simulink model "PUMA_8MM"  (Simulink 8.6)
settings: Solver=ode5  StartTime=0.0  StopTime=3  FixedStep=0.003  RelTol=1e-3
undefined symbols (not defined in the file): magnitude
libraries: vrlib x8, simulink x5
(part 2 of 2)

== matlab function BFT_old/PathFounder_ftk(tau) ==
  data: ksi output double; teta output double; fi output double; w input double; ax output double; ay output double; az output double; bx output double; by output double; bz output double; paramdt output double; paramSUM input double; time input double
function [ksi,teta,fi,ax,ay,az,bx,by,bz,paramdt] = fcn(w,paramSUM,time)

  % reset initial conditions, when -1 change on +1_
  
  % отсчет номера рабочего сплайна_
  num = 2;
  for k = 1:1:20
    if (paramSUM>k) num = k+2; end;
  end;
  param = paramSUM - num + 2;
  
  % =======================================================================
  
  %% задание опорных точек_
  % окружность_
  Pksi  = [0 0 0 0 0 0 0 0 0 0 0 0 0 0 0 0 0 0 0 0];
  Pteta = [0 0 0 0 0 0 0 0 0 0 0 0 0 0 0 0 0 0 0 0]; 
  Pfi   = [0 0 0 0 0 0 0 0 0 0 0 0 0 0 0 0 0 0 0 0];

  d = 0.4;%*1.525;
  b = 0.2*0;
  c = 0.2;
%  % окружность_
%  PN1ksi  = [d 0 -d 0 d 0 -d 0 d 0 -d 0 d 0 -d 0 d 0 -d 0];
%  PN1teta = [0 0 0 0 0 0 0 0 0 0 0 0 0 0 0 0 0 0 0 0];
%  PN1fi   = [0 -d 0 d 0 -d 0 d 0 -d 0 d 0 -d 0 d 0 -d 0 d];
%  PN2ksi  = [d 0 -d 0 d 0 -d 0 d 0 -d 0 d 0 -d 0 d 0 -d 0];
%  PN2teta = [0 0 0 0 0 0 0 0 0 0 0 0 0 0 0 0 0 0 0 0];
%  PN2fi   = [0 -d 0 d 0 -d 0 d 0 -d 0 d 0 -d 0 d 0 -d 0 d]; 

%  PN1ksi  = [0 0 0 0 0 0 0 0 0 0 0 0 0 0 0 0 0 0 0 0];
%  PN1teta = [0 0 0 0 0 0 0 0 0 0 0 0 0 0 0 0 0 0 0 0];
%  PN1fi   = [d -d d -d d -d d -d d -d d -d d -d d -d d -d d -d];
%  PN2ksi  = [0 0 0 0 0 0 0 0 0 0 0 0 0 0 0 0 0 0 0 0];
%  PN2teta = [0 0 0 0 0 0 0 0 0 0 0 0 0 0 0 0 0 0 0 0];
%  PN2fi   = [d -d d -d d -d d -d d -d d -d d -d d -d d -d d -d]; 

%  PN1ksi  = [0 0 0 0 0 0 0 0 0 0 0 0 0 0 0 0 0 0 0 0];
%  PN1teta = [d -d d -d d -d d -d d -d d -d d -d d -d d -d d -d];
%  PN1fi   = [0 0 0 0 0 0 0 0 0 0 0 0 0 0 0 0 0 0 0 0];
%  PN2ksi  = [0 0 0 0 0 0 0 0 0 0 0 0 0 0 0 0 0 0 0 0];
%  PN2teta = [d -d d -d d -d d -d d -d d -d d -d d -d d -d d -d];
%  PN2fi   = [0 0 0 0 0 0 0 0 0 0 0 0 0 0 0 0 0 0 0 0]; 

%  PN1ksi  = [d -d d -d d -d d -d d -d d -d d -d d -d d -d d -d];
%  PN1teta = [0 0 0 0 0 0 0 0 0 0 0 0 0 0 0 0 0 0 0 0];
%  PN1fi   = [0 0 0 0 0 0 0 0 0 0 0 0 0 0 0 0 0 0 0 0];
%  PN2ksi  = [d -d d -d d -d d -d d -d d -d d -d d -d d -d d -d];
%  PN2teta = [0 0 0 0 0 0 0 0 0 0 0 0 0 0 0 0 0 0 0 0];
%  PN2fi   = [0 0 0 0 0 0 0 0 0 0 0 0 0 0 0 0 0 0 0 0]; 

  PN1ksi  = [d -d d -d d -d d -d d -d d -d d -d d -d d -d d -d];
  PN1teta = [c -c c -c c -c c -c c -c c -c c -c c -c c -c c -c];
  PN1fi   = [-b b -b b -b b -b b -b b -b b -b b -b b -b b -b b];
  PN2ksi  = [d -d d -d d -d d -d d -d d -d d -d d -d d -d d -d];
  PN2teta = [c -c c -c c -c c -c c -c c -c c -c c -c c -c c -c];
  PN2fi   = [-b b -b b -b b -b b -b b -b b -b b -b b -b b -b b]; 

  % =======================================================================

  % расчет коэффициентов A,B,C,D_
  Aksi  = -Pksi(num)    + 3*PN1ksi(num)  - 3*PN2ksi(num)  + Pksi(num+1);
  Ateta = -Pteta(num)   + 3*PN1teta(num) - 3*PN2teta(num) + Pteta(num+1);
  Afi   = -Pfi(num)     + 3*PN1fi(num)   - 3*PN2fi(num)   + Pfi(num+1);
  Bksi  = 3*Pksi(num)   - 6*PN1ksi(num)  + 3*PN2ksi(num);
  Bteta = 3*Pteta(num)  - 6*PN1teta(num) + 3*PN2teta(num);
  Bfi   = 3*Pfi(num)    - 6*PN1fi(num)   + 3*PN2fi(num);
  Cksi  = -3*Pksi(num)  + 3*PN1ksi(num);
  Cteta = -3*Pteta(num) + 3*PN1teta(num);
  Cfi   = -3*Pfi(num)   + 3*PN1fi(num);
  Dksi  = Pksi(num);
  Dteta = Pteta(num);
  Dfi   = Pfi(num);
  
  ksi  = Aksi*param^3  + Bksi*param^2  + Cksi*param  + Dksi;
  teta = Ateta*param^3 + Bteta*param^2 + Cteta*param + Dteta;
  fi   = Afi*param^3   + Bfi*param^2   + Cfi*param   + Dfi;
  
ksi  = 0;
teta = 0;
fi   = 0;

  % расчет производной параметрического времени_
  paramdt = w/(  (Aksi*3*param^2+Bksi*2*param+Cksi)^2 + (Ateta*3*param^2+Bteta*2*param+Cteta)^2 + (Afi*3*param^2+Bfi*2*param+Cfi)^2  )^(0.5);

  % =======================================================================
  
  Ea = [ 0 ; 1 ; 0 ];
  Eb = [ 0 ; 0 ; 1 ];
  
  % Mx(ksi) - поворот вокруг оси OX на на угол ksi_
  Mxksi  = [ 1         0          0         ; 0       cos(ksi) (-sin(ksi)) ; 0            sin(ksi) cos(ksi) ];
  Myteta = [ cos(teta) 0          sin(teta) ; 0       1        0           ; (-sin(teta)) 0        cos(teta)];
  Mzfi   = [ cos(fi)   (-sin(fi)) 0         ; sin(fi) cos(fi)  0           ; 0            0        1        ];  
  
  a = Mxksi*Myteta*Mzfi*Ea;
  b = Mxksi*Myteta*Mzfi*Eb;
  
  ax = a(1,1);
  ay = a(2,1);
  az = a(3,1);
  bx = b(1,1);
  by = b(2,1);
  bz = b(3,1);
  
%ax = 0;
%az = 0.2*sin(time*3.141592);
%ay = sqrt(1-az*az);
%bx = 0;
%by = 0.2*sin(time*3.141592);
%bz = sqrt(1-by*by); 

%ax = 0;
%ay = 0;
%az = 1;
%bx = -1;
%by = 0;
%bz = 0;

end

== matlab function BFq7_integrator/OZK_q7+ ==
  data: x input double; y input double; z input double; q7pr output double; ax input double; ay input double; az input double; bx input double; by input double; bz input double; q7 input double; o1 output double; o2 output double; o3 output double
function [q7pr,o1,o2,o3] = fcn(x,y,z,ax,ay,az,bx,by,bz,q7)
   
   % q7 настраивается так, чтобы расстояние W2_cr-W2 было больше Rmin.
 
    pi = 3.14159265358979;
    % Длины звеньев.
    L1 = 0.4;
    L2 = 0.7;
    L3 = 0.7;
    L4 = 0.1;

    % Тестовая надбавка для q7.
    dq = 0.01;
    
    % Ограничения по положению по степеням подвижности i=1,7.
    q1min = -pi/2;    q1max =  pi/2;
    q2min = -pi/2;    q2max =  pi/2;
    q3min = -pi/2;    q3max =  pi/2;
    q4min = -pi/2;    q4max =  pi/2;
    q5min = -pi/2;    q5max =  pi/2;
    q6min = -pi/2;    q6max =  pi/2;
    q7min = -5;       q7max =  5;
    
% =========================================================================    
% ===================== Опред. текущее значение q1-q6 =====================  
% =========================================================================

    rx = x - q7;
    ry = y     ;
    rz = z     ;

    Rx = rx-ax*L4;
    Ry = ry-ay*L4;
    Rz = rz-az*L4;
 
  if (Ry==0) Ry = 0.0000001; end;  
  q1 = -atan(Rx/Ry);
  
    f1 = (Rz-L1)/L3;
    f2 = -L2/L3;
    f3 = Ry/(L3*cos(q1));
    
    g1 = 2*f1*f2;
    g2 = 2*f2*f3;
    g3 = 1-f1*f1-f2*f2-f3*f3;
           
  q2 = asin(g3/sqrt(g1*g1+g2*g2)) - atan(f3/f1); 
    if (q2<-pi/2) q2 = q2+pi; end;
  q3 = asin(f1+f2*sin(q2)) - q2;   
  
    fi  = q2+q3;  
    sfi = sin(fi);
    cfi = cos(fi);
    if (ay==0) ay = 0.0000001; end;  
    alfa = -q1 - atan(ax/ay); 
    if (abs(alfa)<0.0000001) alfa = 0; end;

  if (alfa >= 0) q5 =  acos(-ax*sin(q1)*cfi + ay*cos(q1)*cfi + az*sfi); 
  else           q5 = -acos(-ax*sin(q1)*cfi + ay*cos(q1)*cfi + az*sfi);
  end;                                                                 
  
    k = az - sfi*cos(q5);

  if (q5==0) q5 = 0.0000001; end;
  q4 = acos((-ax*cos(q1)-ay*sin(q1))/sin(q5));
  if (k  < 0) q4 = -q4; end; 
  if (q5 < 0) q4 = -q4; end; 
    
    gammax =  bz*(sin(q1)*sin(q4) - cos(q1)*sfi*cos(q4)) - by*cfi*cos(q4);
    gammay = -bz*(cos(q1)*sin(q4) + sin(q1)*sfi*cos(q4)) + bx*cfi*cos(q4);
    
    betta = gammax*ax + gammay*ay;
    
  q6 = acos(  bx*(cos(q1)*sin(q4)+sin(q1)*sfi*cos(q4))  +  by*(sin(q1)*sin(q4)-cos(q1)*sfi*cos(q4))  +  bz*(cfi*cos(q4))  );
  if (betta<0)  q6 = -q6; end; 
  
% -------------------- Текущее значение maxInd --------------------------

  Ind1  = abs(q1)/q1max;
  Ind2  = abs(q2)/q2max;
  Ind3  = abs(q3)/q3max;
  Ind4  = abs(q4)/q4max;
  Ind5  = abs(q5)/q5max;
  Ind6  = abs(q6)/q6max;
  Ind7  = abs(q7)/q7max;
  Ind8  = ( 2 - sqrt(ax*ax+ay*ay) - sqrt(rx*rx+ry*ry)/(L2+L3+L4) ) / 2;
  Ind9  = ( q5max - abs(q5) )/ q5max;
  Ind10 = ( q3max - abs(q3)/2.5 )/ q3max; % 4.7
  
  J = 0;
  J = max (J,Ind1);
  J = max (J,Ind2);
  J = max (J,Ind3);
  J = max (J,Ind4);
  J = max (J,Ind5);
  J = max (J,Ind6);
  J = max (J,Ind7);
  J = max (J,Ind8);
  J = max (J,Ind9);
  J = max (J,Ind10);

  maxInd = J;
  
% =========================================================================    
% ============================ @'но для q7+dq =============================  
% ========================================================================= 

    rx = x - (q7+dq);
    ry = y          ;
    rz = z          ;

    Rx = rx-ax*L4;
    Ry = ry-ay*L4;
    Rz = rz-az*L4;
 
  if (Ry==0) Ry = 0.0000001; end;  
  q1 = -atan(Rx/Ry);
  
    f1 = (Rz-L1)/L3;
    f2 = -L2/L3;
    f3 = Ry/(L3*cos(q1));
    
    g1 = 2*f1*f2;
    g2 = 2*f2*f3;
    g3 = 1-f1*f1-f2*f2-f3*f3;
           
  q2 = asin(g3/sqrt(g1*g1+g2*g2)) - atan(f3/f1); 
    if (q2<-pi/2) q2 = q2+pi; end;
  q3 = asin(f1+f2*sin(q2)) - q2;   
  
    fi  = q2+q3;  
    sfi = sin(fi);
    cfi = cos(fi);
    if (ay==0) ay = 0.0000001; end;  
    alfa = -q1 - atan(ax/ay); 
    if (abs(alfa)<0.0000001) alfa = 0; end;

  if (alfa >= 0) q5 =  acos(-ax*sin(q1)*cfi + ay*cos(q1)*cfi + az*sfi); 
  else           q5 = -acos(-ax*sin(q1)*cfi + ay*cos(q1)*cfi + az*sfi);
  end;                                                                 
  
    k = az - sfi*cos(q5);

  if (q5==0) q5 = 0.0000001; end;
  q4 = acos((-ax*cos(q1)-ay*sin(q1))/sin(q5));
  if (k  < 0) q4 = -q4; end; 
  if (q5 < 0) q4 = -q4; end; 
    
    gammax =  bz*(sin(q1)*sin(q4) - cos(q1)*sfi*cos(q4)) - by*cfi*cos(q4);
    gammay = -bz*(cos(q1)*sin(q4) + sin(q1)*sfi*cos(q4)) + bx*cfi*cos(q4);
    
    betta = gammax*ax + gammay*ay;
    
  q6 = acos(  bx*(cos(q1)*sin(q4)+sin(q1)*sfi*cos(q4))  +  by*(sin(q1)*sin(q4)-cos(q1)*sfi*cos(q4))  +  bz*(cfi*cos(q4))  );
  if (betta<0)  q6 = -q6; end; 
  
% -------------------- Текущее значение maxInd(q7+dq7) --------------------

  Ind1  = abs(q1)/q1max;
  Ind2  = abs(q2)/q2max;
  Ind3  = abs(q3)/q3max;
  Ind4  = abs(q4)/q4max;
  Ind5  = abs(q5)/q5max;
  Ind6  = abs(q6)/q6max;
  Ind7  = abs(q7)/q7max;
  Ind8  = ( 2 - sqrt(ax*ax+ay*ay) - sqrt(rx*rx+ry*ry)/(L2+L3+L4) ) / 2;
  Ind9  = ( q5max - abs(q5) )/ q5max;
  Ind10 = ( q3max - abs(q3)/2.5 )/ q3max; % 4.7
  
  J = 0;
  J = max (J,Ind1);
  J = max (J,Ind2);
  J = max (J,Ind3);
  J = max (J,Ind4);
  J = max (J,Ind5);
  J = max (J,Ind6);
  J = max (J,Ind7);
  J = max (J,Ind8);
  J = max (J,Ind9);
  J = max (J,Ind10);

  maxIndp = J;
         
% =========================================================================    
% ============================ @'но для q7-dq =============================   
% =========================================================================
   
    rx = x - (q7-dq);
    ry = y          ;
    rz = z          ;

    Rx = rx-ax*L4;
    Ry = ry-ay*L4;
    Rz = rz-az*L4;
 
  if (Ry==0) Ry = 0.0000001; end;  
  q1 = -atan(Rx/Ry);
  
    f1 = (Rz-L1)/L3;
    f2 = -L2/L3;
    f3 = Ry/(L3*cos(q1));
    
    g1 = 2*f1*f2;
    g2 = 2*f2*f3;
    g3 = 1-f1*f1-f2*f2-f3*f3;
           
  q2 = asin(g3/sqrt(g1*g1+g2*g2)) - atan(f3/f1); 
    if (q2<-pi/2) q2 = q2+pi; end;
  q3 = asin(f1+f2*sin(q2)) - q2;   
  
    fi  = q2+q3;  
    sfi = sin(fi);
    cfi = cos(fi);
    if (ay==0) ay = 0.0000001; end;  
    alfa = -q1 - atan(ax/ay); 
    if (abs(alfa)<0.0000001) alfa = 0; end;

  if (alfa >= 0) q5 =  acos(-ax*sin(q1)*cfi + ay*cos(q1)*cfi + az*sfi); 
  else           q5 = -acos(-ax*sin(q1)*cfi + ay*cos(q1)*cfi + az*sfi);
  end;                                                                 
  
    k = az - sfi*cos(q5);

  if (q5==0) q5 = 0.00001; end;
  q4 = acos((-ax*cos(q1)-ay*sin(q1))/sin(q5));
  if (k  < 0) q4 = -q4; end; 
  if (q5 < 0) q4 = -q4; end; 
    
    gammax =  bz*(sin(q1)*sin(q4) - cos(q1)*sfi*cos(q4)) - by*cfi*cos(q4);
    gammay = -bz*(cos(q1)*sin(q4) + sin(q1)*sfi*cos(q4)) + bx*cfi*cos(q4);
    
    betta = gammax*ax + gammay*ay;
    
  q6 = acos(  bx*(cos(q1)*sin(q4)+sin(q1)*sfi*cos(q4))  +  by*(sin(q1)*sin(q4)-cos(q1)*sfi*cos(q4))  +  bz*(cfi*cos(q4))  );
  if (betta<0)  q6 = -q6; end; 
  
% -------------------- Текущее значение maxInd(q7-dq7) --------------------

  Ind1  = abs(q1)/q1max;
  Ind2  = abs(q2)/q2max;
  Ind3  = abs(q3)/q3max;
  Ind4  = abs(q4)/q4max;
  Ind5  = abs(q5)/q5max;
  Ind6  = abs(q6)/q6max;
  Ind7  = abs(q7)/q7max;
  Ind8  = ( 2 - sqrt(ax*ax+ay*ay) - sqrt(rx*rx+ry*ry)/(L2+L3+L4) ) / 2;
  Ind9  = ( q5max - abs(q5) )/ q5max;
  Ind10 = ( q3max - abs(q3)/2.5 )/ q3max; % 4.7
  
  J = 0;
  J = max (J,Ind1);
  J = max (J,Ind2);
  J = max (J,Ind3);
  J = max (J,Ind4);
  J = max (J,Ind5);
  J = max (J,Ind6);
  J = max (J,Ind7);
  J = max (J,Ind8);
  J = max (J,Ind9);
  J = max (J,Ind10);

  maxIndn = J;
  
% =========================================================================    
% ============================= Выбор q7pr +/- ============================  
% =========================================================================  

  % q7pr - фиксированная скорость перемещения основания робота. 
  q7pr = 0.3;
  % Indth - пороговое значение максимального индикатора. 
  Indth = 0.9;

  if (maxIndn<maxIndp) q7pr = -q7pr; end;
  if (maxInd <Indth)   q7pr = 0;     end;

  o1 = maxInd;
  o2 = maxIndp;
  o3 = maxIndn;
  
end

== matlab function BFT_old/PathFounder_xyz(tau) ==
  data: v input double; x output double; y output double; z output double; num output double; paramdt output double; paramSUM input double
function [x,y,z,num,paramdt] = fcn(v,paramSUM)

  % reset initial conditions, when -1 change on +1.
  
  % Отсчет номера рабочего сплайна.
  num = 2;
  for k = 1:1:99
    if (paramSUM>k) num = k+2; end;
  end;
  param = paramSUM - num + 2;
  
  L1 = 0.4;
  L2 = 0.7;
  L3 = 0.7;
  L4 = 0.1;  
  
  % =======================================================================
  
  %% Окружность 0.4R с центром в (.)(0;ky;kz), наклоненная в пространстве.
%  ky = 1.1;   % смещение по оси оу.                                    
%  kz = 0.5;   % смещение по оси оz.
%  R  = 0.35;  % радиус окружности. 
%  fi = -0.2;  % угол наклона окружности.
%    dy00 = 0; % смещения окружности по оси оу.
%    dy05 = 0.5*R*sin(-fi); 
%    dy10 = 1.0*R*sin(-fi);
%    dy15 = 1.5*R*sin(-fi);
%    dy20 = 2.0*R*sin(-fi);
%  Px = [0       R       0       -R      0       R       0       -R      0       R       0       -R      0       R       0       -R      0       R       0       -R      ];
%  Py = [ky+dy00 ky+dy10 ky+dy20 ky+dy10 ky+dy00 ky+dy10 ky+dy20 ky+dy10 ky+dy00 ky+dy10 ky+dy20 ky+dy10 ky+dy00 ky+dy10 ky+dy20 ky+dy10 ky+dy00 ky+dy10 ky+dy20 ky+dy10 ]; 
%  Pz = [kz-R    kz      kz+R    kz      kz-R    kz      kz+R    kz      kz-R    kz      kz+R    kz      kz-R    kz      kz+R    kz      kz-R    kz      kz+R    kz      ];
  % Направляющие.
%  d = 0.02075*R/0.4;
%  PN1x = [R/2+d    R        -R/2-d    -R       R/2+d    R        -R/2-d    -R       R/2+d    R        -R/2-d    -R       R/2+d    R        -R/2-d    -R       R/2+d    R        -R/2-d    -R       ];
%  PN1y = [ky+dy00  ky+dy15  ky+dy20   ky+dy05  ky+dy00  ky+dy15  ky+dy20   ky+dy05  ky+dy00  ky+dy15  ky+dy20   ky+dy05  ky+dy00  ky+dy15  ky+dy20   ky+dy05  ky+dy00  ky+dy15  ky+dy20   ky+dy05  ];
%  PN1z = [kz-R     kz+R/2+d kz+R      kz-R/2-d kz-R     kz+R/2+d kz+R      kz-R/2-d kz-R     kz+R/2+d kz+R      kz-R/2-d kz-R     kz+R/2+d kz+R      kz-R/2-d kz-R     kz+R/2+d kz+R      kz-R/2-d ];
%  PN2x = [R        R/2+d    -R        -R/2-d   R        R/2+d    -R        -R/2-d   R        R/2+d    -R        -R/2-d   R        R/2+d    -R        -R/2-d   R        R/2+d    -R        -R/2-d   ];
%  PN2y = [ky+dy05  ky+dy20  ky+dy15   ky+dy00  ky+dy05  ky+dy20  ky+dy15   ky+dy00  ky+dy05  ky+dy20  ky+dy15   ky+dy00  ky+dy05  ky+dy20  ky+dy15   ky+dy00  ky+dy05  ky+dy20  ky+dy15   ky+dy00  ];
%  PN2z = [kz-R/2-d kz+R     kz+R/2+d  kz-R     kz-R/2-d kz+R     kz+R/2+d  kz-R     kz-R/2-d kz+R     kz+R/2+d  kz-R     kz-R/2-d kz+R     kz+R/2+d  kz-R     kz-R/2-d kz+R     kz+R/2+d  kz-R     ]; 

  %% Синусоида y=A*sin(...)+c
%  A  = 0.05;  % амплитуда в плоскости OXY.
%  B  = 0.25;  % амплитуда в плоскости OXZ.
%  c  = 1.2;   % смещение по оси OY.
%  k  = 0.4;   % смещение по оси OZ.
%  L  = 0.15;  % растягивание по OX.
%  Px = [-4*L -3*L  -2*L  -1*L   0*L   1*L   2*L   3*L   4*L   5*L   6*L   7*L   8*L   9*L   10*L  11*L  12*L  13*L  14*L  15*L ];
%  Py = [c    c     c     c      c     c     c     c     c     c     c     c     c     c     c     c     c     c     c     c    ];
%  Pz = [k    k     k     k      k     k     k     k     k     k     k     k     k     k     k     k     k     k     k     k    ];    
  % Направляющие.
%  d = 0.05;  % смещение направляющих.
%  PN1x = [-4*L+d -3*L+d -2*L+d -1*L+d 0*L+d 1*L+d 2*L+d 3*L+d 4*L+d 5*L+d 6*L+d 7*L+d 8*L+d 9*L+d  10*L+d 11*L+d 12*L+d 13*L+d 14*L+d 15*L+d];
%  PN1y = [c+A    c-A    c+A    c-A    c+A   c-A   c+A   c-A   c+A   c-A   c+A   c-A   c+A   c-A    c+A    c-A    c+A    c-A    c+A    c-A   ];
%  PN1z = [k+B    k-B    k+B    k-B    k+B   k-B   k+B   k-B   k+B   k-B   k+B   k-B   k+B   k-B    k+B    k-B    k+B    k-B    k+B    k-B   ]; 
%  PN2x = [-3*L-d -2*L-d -1*L-d 0*L-d  1*L-d 2*L-d 3*L-d 4*L-d 5*L-d 6*L-d 7*L-d 8*L-d 9*L-d 10*L-d 11*L-d 12*L-d 13*L-d 14*L-d 15*L-d 16*L-d];
%  PN2y = [c+A    c-A    c+A    c-A    c+A   c-A   c+A   c-A   c+A   c-A   c+A   c-A   c+A   c-A    c+A    c-A    c+A    c-A    c+A    c-A   ];
%  PN2z = [k+B    k-B    k+B    k-B    k+B   k-B   k+B   k-B   k+B   k-B   k+B   k-B   k+B   k-B    k+B    k-B    k+B    k-B    k+B    k-B   ];  

  %% Кривая, поднимающейся снизу вверх по поверхности цилиндра радиусом R и высотой H. 
  %   важны только первые 5 сплайнов.
%  R = 0.7;  % радиус цилиндра.
%  H = 0.25; % коэффициент высоты цилиндра.
%  Px = [0*R  1*R 0*R -1*R 0*R  0*R  1*R 0*R -1*R 0*R  0*R  1*R 0*R -1*R 0*R  0*R  1*R 0*R -1*R 0*R  ];
%  Py = [-1*R 0*R 1*R 0*R  -1*R -1*R 0*R 1*R 0*R  -1*R -1*R 0*R 1*R 0*R  -1*R -1*R 0*R 1*R 0*R  -1*R ]; 
%  Pz = [-1*H 0*H 1*H 2*H  3*H  -1*H 0*H 1*H 2*H  3*H  -1*H 0*H 1*H 2*H  3*H  -1*H 0*H 1*H 2*H  3*H  ];   
  % Направляющие.
%  d = 0.02075*2.5*R;
%  PN1x = [0.5*R+d     1*R        -0.5*R-d   -1*R      0.5*R+d     0.5*R+d     1*R        -0.5*R-d   -1*R      0.5*R+d     0.5*R+d     1*R        -0.5*R-d   -1*R      0.5*R+d     0.5*R+d     1*R        -0.5*R-d   -1*R      0.5*R+d     ];
%  PN1y = [-1*R        0.5*R+d    1*R        -0.5*R-d  -1*R        -1*R        0.5*R+d    1*R        -0.5*R-d  -1*R        -1*R        0.5*R+d    1*R        -0.5*R-d  -1*R        -1*R        0.5*R+d    1*R        -0.5*R-d  -1*R        ];
%  PN1z = [-0.75*H+d/5 0.25*H+d/5 1.25*H+d/5 2.25*H+d/5 3.25*H+d/5 -0.75*H+d/5 0.25*H+d/5 1.25*H+d/5 2.25*H+d/5 3.25*H+d/5 -0.75*H+d/5 0.25*H+d/5 1.25*H+d/5 2.25*H+d/5 3.25*H+d/5 -0.75*H+d/5 0.25*H+d/5 1.25*H+d/5 2.25*H+d/5 3.25*H+d/5 ];
%  PN2x = [1*R         0.5*R+d    -1*R       -0.5*R-d  1*R         1*R         0.5*R+d    -1*R       -0.5*R-d  1*R         1*R         0.5*R+d    -1*R       -0.5*R-d  1*R         1*R         0.5*R+d    -1*R       -0.5*R-d  1*R         ];
%  PN2y = [-0.5*R-d    1*R        0.5*R+d    -1*R      -0.5*R-d    -0.5*R-d    1*R        0.5*R+d    -1*R      -0.5*R-d    -0.5*R-d    1*R        0.5*R+d    -1*R      -0.5*R-d    -0.5*R-d    1*R        0.5*R+d    -1*R      -0.5*R-d    ];
%  PN2z = [-0.25*H-d/5 0.75*H-d/5 1.75*H-d/5 2.75*H-d/5 3.75*H-d/5 -0.25*H-d/5 0.75*H-d/5 1.75*H-d/5 2.75*H-d/5 3.75*H-d/5 -0.25*H-d/5 0.75*H-d/5 1.75*H-d/5 2.75*H-d/5 3.75*H-d/5 -0.25*H-d/5 0.75*H-d/5 1.75*H-d/5 2.75*H-d/5 3.75*H-d/5 ]; 

  %% Прямая, параллельная oz, проходящая через (X;Y;Z).
%  X = 0;
%  Y = 1.1;
%  Z = 1;
%  Px = [X   X      X     X      X   X   X      X     X      X   X   X      X     X      X   X   X      X     X      X   ];
%  Py = [Y   Y      Y     Y      Y   Y   Y      Y     Y      Y   Y   Y      Y     Y      Y   Y   Y      Y     Y      Y   ];
%  Pz = [1*Z 0.75*Z 0.5*Z 0.25*Z 0*Z 1*Z 0.75*Z 0.5*Z 0.25*Z 0*Z 1*Z 0.75*Z 0.5*Z 0.25*Z 0*Z 1*Z 0.75*Z 0.5*Z 0.25*Z 0*Z ]; 
  % Направляющие.
%  PN1x = [X      X      X      X      X       X      X      X      X      X       X      X      X      X      X       X      X      X      X      X       ];
%  PN1y = [Y      Y      Y      Y      Y       Y      Y      Y      Y      Y       Y      Y      Y      Y      Y       Y      Y      Y      Y      Y       ];
%  PN1z = [0.95*Z 0.70*Z 0.45*Z 0.20*Z -0.05*Z 0.95*Z 0.70*Z 0.45*Z 0.20*Z -0.05*Z 0.95*Z 0.70*Z 0.45*Z 0.20*Z -0.05*Z 0.95*Z 0.70*Z 0.45*Z 0.20*Z -0.05*Z ];
%  PN2x = [X      X      X      X      X       X      X      X      X      X       X      X      X      X      X       X      X      X      X      X       ];
%  PN2y = [Y      Y      Y      Y      Y       Y      Y      Y      Y      Y       Y      Y      Y      Y      Y       Y      Y      Y      Y      Y       ];
%  PN2z = [0.80*Z 0.55*Z 0.30*Z 0.05*Z -0.20*Z 0.80*Z 0.55*Z 0.30*Z 0.05*Z -0.20*Z 0.80*Z 0.55*Z 0.30*Z 0.05*Z -0.20*Z 0.80*Z 0.55*Z 0.30*Z 0.05*Z -0.20*Z ];

  %% Эллипс. Поперечные сечения - L и W.
%  L = 0.5;
%  W = 2;
%  Px = [-L L -L L -L L -L L -L L -L L -L L -L L -L L -L L];
%  Py = [0  0 0  0 0  0 0  0 0  0 0  0 0  0 0  0 0  0 0  0]; 
%  Pz = [0  0 0  0 0  0 0  0 0  0 0  0 0  0 0  0 0  0 0  0];  
  % Направляющие.
%  PN1x = [-L L  -L L  -L L  -L L  -L L  -L L  -L L  -L L  -L L  -L L ];
%  PN1y = [W  -W W  -W W  -W W  -W W  -W W  -W W  -W W  -W W  -W W  -W];
%  PN1z = [0  0  0  0  0  0  0  0  0  0  0  0  0  0  0  0  0  0  0  0 ];
%  PN2x = [L  -L L  -L L  -L L  -L L  -L L  -L L  -L L  -L L  -L L  -L];
%  PN2y = [W  -W W  -W W  -W W  -W W  -W W  -W W  -W W  -W W  -W W  -W];
%  PN2z = [0  0  0  0  0  0  0  0  0  0  0  0  0  0  0  0  0  0  0  0 ];

  %% Хитрые спирали.
%  L = 0.15;   % растягивание по ox.
%  H = 1.1;    % смещение по oy.
%  J = 0.25;   % смещение по oz.
%  M = 0.3;    % ширина петель.
%  k = 0.2;    % растягивание петель.
%  Px = [-4*L -3*L  -2*L  -1*L   0*L   1*L   2*L   3*L   4*L   5*L   6*L   7*L   8*L   9*L   10*L  11*L  12*L  13*L  14*L  15*L ];
%  Py = [H     H     H     H     H     H     H     H     H     H     H     H     H     H     H     H     H     H     H     H    ];
%  Pz = [J     J     J     J     J     J     J     J     J     J     J     J     J     J     J     J     J     J     J     J    ]; 
  % Направляющие.
%  PN1x = [-3*L+k  -2*L+k  -1*L+k  0*L+k   1*L+k   2*L+k   3*L+k   4*L+k   5*L+k   6*L+k   7*L+k   8*L+k   9*L+k   10*L+k  11*L+k  12*L+k  13*L+k  14*L+k  15*L+k  16*L+k  ];
%  PN1y = [H       H       H       H       H       H       H       H       H       H       H       H       H       H       H       H       H       H       H       H       ];
%  PN1z = [J+M     J-M     J+M     J-M     J+M     J-M     J+M     J-M     J+M     J-M     J+M     J-M     J+M     J-M     J+M     J-M     J+M     J-M     J+M     J-M     ];
%  PN2x = [-4*L-k  -3*L-k  -2*L-k  -1*L-k  0*L-k   1*L-k   2*L-k   3*L-k   4*L-k   5*L-k   6*L-k   7*L-k   8*L-k   9*L-k   10*L-k  11*L-k  12*L-k  13*L-k  14*L-k  15*L-k  ];
%  PN2y = [H       H       H       H       H       H       H       H       H       H       H       H       H       H       H       H       H       H       H       H       ];
%  PN2z = [J+M     J-M     J+M     J-M     J+M     J-M     J+M     J-M     J+M     J-M     J+M     J-M     J+M     J-M     J+M     J-M     J+M     J-M     J+M     J-M     ];

  %% Прямая, параллельная ox, проходящая через (X;Y;Z).
%  X  = 0.3;
%  Y  = L2*cos(pi/6)+L3+L4*0.97;
%  Z  = L1+L2*sin(pi/6);
%  Px = [-1*X -0.75*X -0.5*X -0.25*X 0*X 0.25*X 0.5*X 0.75*X 1*X 0.75*X 0.5*X 0.25*X 0*X -0.25*X -0.5*X -0.75*X -1*X -0.75*X -0.5*X -0.25*X ];
%  Py = [Y    Y       Y      Y       Y   Y      Y     Y      Y   Y      Y     Y      Y   Y       Y      Y       Y    Y       Y      Y       ];
%  Pz = [Z    Z       Z      Z       Z   Z      Z     Z      Z   Z      Z     Z      Z   Z       Z      Z       Z    Z       Z      Z       ];
  % Направляющие.
%  PN1x = [-0.9*X -0.7*X -0.4*X -0.2*X 0.1*X  0.3*X 0.6*X 0.8*X 0.9*X 0.7*X 0.4*X 0.2*X -0.1*X -0.3*X -0.6*X -0.8*X -0.9*X -0.7*X -0.4*X -0.2*X ];
%  PN1y = [Y      Y      Y      Y      Y      Y     Y     Y     Y     Y     Y     Y     Y      Y      Y      Y      Y      Y      Y      Y      ];
%  PN1z = [Z      Z      Z      Z      Z      Z     Z     Z     Z     Z     Z     Z     Z      Z      Z      Z      Z      Z      Z      Z      ];
%  PN2x = [-0.8*X -0.6*X -0.3*X -0.1*X 0.2*X  0.4*X 0.7*X 0.9*X 0.8*X 0.6*X 0.3*X 0.1*X -0.2*X -0.4*X -0.7*X -0.9*X -0.8*X -0.6*X -0.3*X -0.1*X ];
%  PN2y = [Y      Y      Y      Y      Y      Y     Y     Y     Y     Y     Y     Y     Y      Y      Y      Y      Y      Y      Y      Y      ];
%  PN2z = [Z      Z      Z      Z      Z      Z     Z     Z     Z     Z     Z     Z     Z      Z      Z      Z      Z      Z      Z      Z      ];

  %% Окружность 0.4R с центром в (.)(0;ky;kz) и хитрые спирали.
  ky = 1.1;       % Окружность: смещение по оси оу.                                    
  kz = 0.5;       % Окружность: смещение по оси оz.
  R  = 0.3;       % Окружность: радиус окружности.
  d  = 0.03*R;    % Окружность: растягивание направляющих.
  H  = 1.1;       % Спирали:    смещение по oy.
  J  = 0.25;      % Спирали:    смещение по oz.
  L  = 0.07;      % Спирали:    ширина петель по ox.
  k  = 0.2;       % Спирали:    высота петель по oz.
  e  = 0.12;      % Спирали:    расшерение петель по ох.
  Y  = (L2*cos(pi/6)+L3+L4)*0.995; % Точка сингулярности №2.
  Z  = (L1+L2*sin(pi/6))   *0.995; % Точка сингулярности №2.
 
  Px   = [-R  0     R   0     -R                                    -3*L    -1*L    0    1*L    3*L                       R   0     -R    0     R   0     -R  0     R   0     -R];
  Py   = [ky  ky    ky  ky    ky                                    H       H       Y    H      H                         ky  ky    ky    ky    ky  ky    ky  ky    ky  ky    ky]; 
  Pz   = [kz  kz-R  kz  kz+R  kz                                    J       J       Z    J      J                         kz  kz+R  kz    kz-R  kz  kz+R  kz  kz-R  kz  kz+R  kz];
  % Направляющие.
  PN1x = [-R        R/2+d     R         -R/2-d    -R                -1*L+e  1*L+e  -1*L    3*L+e  4*L+e/2                 R         -R/2-d    -R        R/2+d     R         -R/2-d    -R        R/2+d     R         -R/2-d    -R        ];
  PN1y = [ky        ky        ky        ky        ky                H       H      Y       H      H                       ky        ky        ky        ky        ky        ky        ky        ky        ky        ky        ky        ];
  PN1z = [kz-R/2-d  kz-R      kz+R/2+d  kz+R      kz-k/4            J-k     J+k    Z       J-k    J+k/2                   kz+R/2+d  kz+R      kz-R/2-d  kz-R      kz+R/2+d  kz+R      kz-R/2-d  kz-R      kz+R/2+d  kz+R      kz-R/2-d  ];
  PN2x = [-R/2-d    R         R/2-d     -R        -4*L-e/2          -3*L-e  1*L    -1*L-e  1*L-e  R                       R/2-d     -R        -R/2-d    R         R/2-d     -R        -R/2-d    R         R/2-d     -R        -R/2-d    ];
  PN2y = [ky        ky        ky        ky        ky                H       Y      H       H      H                       ky        ky        ky        ky        ky        ky        ky        ky        ky        ky        ky        ];
  PN2z = [kz-R      kz-R/2-d  kz+R      kz+R/2+d  J+k/2             J-k     Z      J+k     J-k    kz-k/4                  kz+R      kz+R/2+d  kz-R      kz-R/2-d  kz+R      kz+R/2+d  kz-R      kz-R/2-d  kz+R      kz+R/2+d  kz-R      ]; 

%Px   = 1.5*Px;
%PN1x = 1.5*PN1x;
%PN2x = 1.5*PN2x;
  
  %% Траектория для демонстрации первого сингулярного положения.  

  % singular point.
%  alfa  = 1.3;
%  betta = 0;  
%  kx0    =    cos(alfa)*sin(betta)*(L2+L3);
%  ky0    =    cos(alfa)*cos(betta)*(L2+L3); % смещение траектории по оси oz.
%  kz0    = L1+sin(alfa)           *(L2+L3)+L4;
  % удаленная точка.
%  alfa  = 0.9;
%  betta = 0;  
%  kx2    =    cos(alfa)*sin(betta)*(L2+L3);
%  ky2    =    cos(alfa)*cos(betta)*(L2+L3); % смещение траектории по оси oz.
%  kz2    = L1+sin(alfa)           *(L2+L3)+L4;
  % боковые точки (+/-kx).
%  alfa  = 1;
%  betta = 0.3;  
%  kx1    =    cos(alfa)*sin(betta)*(L2+L3);
%  ky1    =    cos(alfa)*cos(betta)*(L2+L3); % смещение траектории по оси oz.
%  kz1    = L1+sin(alfa)           *(L2+L3)+L4;
%  alfa  = 1;
%  betta = -0.3;
%  kx3    =    cos(alfa)*sin(betta)*(L2+L3);
%  ky3    =    cos(alfa)*cos(betta)*(L2+L3); % смещение траектории по оси oz.
%  kz3    = L1+sin(alfa)           *(L2+L3)+L4;
  
%  Px   = [kx0 kx1 kx2 kx3 kx0 kx1 kx2 kx3 kx0 kx1 kx2 kx3 kx0 kx1 kx2 kx3 kx0 kx1 kx2 kx3 ];
%  Py   = [ky0 ky1 ky2 ky3 ky0 ky1 ky2 ky3 ky0 ky1 ky2 ky3 ky0 ky1 ky2 ky3 ky0 ky1 ky2 ky3 ];
%  Pz   = [kz0 kz1 kz2 kz3 kz0 kz1 kz2 kz3 kz0 kz1 kz2 kz3 kz0 kz1 kz2 kz3 kz0 kz1 kz2 kz3 ];
  % Направляющие.
%  PN1x = [(Px(1)+Px(2))/2  (Px(2)+Px(3))/2  (Px(3)+Px(4))/2  (Px(4)+Px(5))/2  (Px(1)+Px(2))/2  (Px(2)+Px(3))/2  (Px(3)+Px(4))/2  (Px(4)+Px(5))/2  ];
%  PN1y = [(Py(1)+Py(2))/2  (Py(2)+Py(3))/2  (Py(3)+Py(4))/2  (Py(4)+Py(5))/2  (Py(1)+Py(2))/2  (Py(2)+Py(3))/2  (Py(3)+Py(4))/2  (Py(4)+Py(5))/2  ];
%  PN1z = [(Pz(1)+Pz(2))/2  (Pz(2)+Pz(3))/2  (Pz(3)+Pz(4))/2  (Pz(4)+Pz(5))/2  (Pz(1)+Pz(2))/2  (Pz(2)+Pz(3))/2  (Pz(3)+Pz(4))/2  (Pz(4)+Pz(5))/2  ];
%  PN2x = [(Px(1)+Px(2))/2  (Px(2)+Px(3))/2  (Px(3)+Px(4))/2  (Px(4)+Px(5))/2  (Px(1)+Px(2))/2  (Px(2)+Px(3))/2  (Px(3)+Px(4))/2  (Px(4)+Px(5))/2  ];
%  PN2y = [(Py(1)+Py(2))/2  (Py(2)+Py(3))/2  (Py(3)+Py(4))/2  (Py(4)+Py(5))/2  (Py(1)+Py(2))/2  (Py(2)+Py(3))/2  (Py(3)+Py(4))/2  (Py(4)+Py(5))/2  ];
%  PN2z = [(Pz(1)+Pz(2))/2  (Pz(2)+Pz(3))/2  (Pz(3)+Pz(4))/2  (Pz(4)+Pz(5))/2  (Pz(1)+Pz(2))/2  (Pz(2)+Pz(3))/2  (Pz(3)+Pz(4))/2  (Pz(4)+Pz(5))/2  ];
  
  %% =======================================================================

  % расчет коэффициентов A,B,C,D_
  Ax = -Px(num) + 3*PN1x(num) - 3*PN2x(num) + Px(num+1);
  Ay = -Py(num) + 3*PN1y(num) - 3*PN2y(num) + Py(num+1);
  Az = -Pz(num) + 3*PN1z(num) - 3*PN2z(num) + Pz(num+1);
  Bx = 3*Px(num) - 6*PN1x(num) + 3*PN2x(num);
  By = 3*Py(num) - 6*PN1y(num) + 3*PN2y(num);
  Bz = 3*Pz(num) - 6*PN1z(num) + 3*PN2z(num);
  Cx = -3*Px(num) + 3*PN1x(num);
  Cy = -3*Py(num) + 3*PN1y(num);
  Cz = -3*Pz(num) + 3*PN1z(num);
  Dx = Px(num);
  Dy = Py(num);
  Dz = Pz(num);
  
  x = Ax*param^3 + Bx*param^2 + Cx*param + Dx;
  y = Ay*param^3 + By*param^2 + Cy*param + Dy;
  z = Az*param^3 + Bz*param^2 + Cz*param + Dz;

  % расчет производной параметрического времени_
  paramdt = v/(  (Ax*3*param^2+Bx*2*param+Cx)^2 + (Ay*3*param^2+By*2*param+Cy)^2 + (Az*3*param^2+Bz*2*param+Cz)^2  )^(0.5);

end

== matlab function MAPcalc/OZK_q7+ ==
  data: x input double; y input double; z input double; ax input double; ay input double; az input double; bx input double; by input double; bz input double; M2 output double; M3 output double; M4 output double; M5 output double; M6 output double; M7 output double; M8 output double; M9 output double; M10 output double; M11 output double; M12 output double; M13 output double; M14 output double; M15 output double; M16 output double; M17 output double; M18 output double; M19 output double; M20 output double; M21 output double; M22 output double; M23 output double; M24 output double; M25 output double; M26 output double; M27 output double; M28 output double; M29 output double; M30 output double; M31 output double; M32 output double; M33 output double; M34 output double; M35 output double; M36 output double; M37 output double; M38 output double; M39 output double; M40 output double
function [M2,M3,M4,M5,M6,M7,M8,M9,M10,M11,M12,M13,M14,M15,M16,M17,M18,M19,M20,M21,M22,M23,M24,M25,M26,M27,M28,M29,M30,M31,M32,M33,M34,M35,M36,M37,M38,M39,M40] = fcn(x,y,z,ax,ay,az,bx,by,bz)
 
    pi = 3.14159265358979;
    N  = 40;
    J  = 0;
    
    MAP = [0 0 0 0 0 0 0 0 0 0 0 0 0 0 0 0 0 0 0 0 0 0 0 0 0 0 0 0 0 0 0 0 0 0 0 0 0 0 0 0];
    for i=1:N, MAP(i) = 999; end;
    
    % Длины звеньев.
    L1 = 0.4;
    L2 = 0.7;
    L3 = 0.7;
    L4 = 0.1;
 
    % Ограничения по положению по степеням подвижности i=1,6.
    q1min = -pi/2;    q1max =  pi/2;
    q2min = -pi/2;    q2max =  pi/2;
    q3min = -pi/2;    q3max =  pi/2;
    q4min = -pi/2;    q4max =  pi/2;
    q5min = -pi/2;    q5max =  pi/2;
    q6min = -pi/2;    q6max =  pi/2;
    q7min = -1;       q7max =  1;
    
    q7 = q7min;
    
% =========================================================================    
% ===================== Опред. текущее значение q1-q6 =====================  
% =========================================================================
 
for i=1:1:N
    
    rx = x - q7;
    ry = y     ;
    rz = z     ;
  
    Rx = rx-ax*L4;
    Ry = ry-ay*L4;
    Rz = rz-az*L4;
 
  if (Ry==0) Ry = 0.0000001; end;  
  q1 = -atan(Rx/Ry);
    if (imag(q1)~=0)                %!
      MAP(i) = 1;                   %!
      if (i == N) q7 = q7min; end;  %!
      q7 = q7 + (q7max-q7min)/N;    %!
      continue;                     %!
    end;                            %!
  
    f1 = (Rz-L1)/L3;
    f2 = -L2/L3;
    f3 = Ry/(L3*cos(q1));
    
    g1 = 2*f1*f2;
    g2 = 2*f2*f3;
    g3 = 1-f1*f1-f2*f2-f3*f3;
    argq2 = g3/sqrt(g1*g1+g2*g2);
    if ((argq2<-1)||(argq2>1))      %!
      MAP(i) = 1;                   %!
      if (i == N) q7 = q7min; end;  %!
      q7 = q7 + (q7max-q7min)/N;    %!
      continue;                     %!
    end;                            %!  
  q2 = asin(argq2) - atan(f3/f1); 
    if (q2<-pi/2) q2 = q2+pi; end;
  q3 = asin(f1+f2*sin(q2)) - q2;   
  
    fi  = q2+q3;  
    sfi = sin(fi);
    cfi = cos(fi);
    if (ay==0) ay = 0.0000001; end;  
    alfa = -q1 - atan(ax/ay); 
    if (abs(alfa)<0.0000001) alfa = 0; end;
 
  if (alfa >= 0) q5 =  acos(-ax*sin(q1)*cfi + ay*cos(q1)*cfi + az*sfi); 
  else           q5 = -acos(-ax*sin(q1)*cfi + ay*cos(q1)*cfi + az*sfi);
  end;                                                                 
  
    k = az - sfi*cos(q5);
 
  if (q5==0) q5 = 0.0000001; end;
  q4 = acos((-ax*cos(q1)-ay*sin(q1))/sin(q5));
  if (k  < 0) q4 = -q4; end; 
  if (q5 < 0) q4 = -q4; end; 
    
    gammax =  bz*(sin(q1)*sin(q4) - cos(q1)*sfi*cos(q4)) - by*cfi*cos(q4);
    gammay = -bz*(cos(q1)*sin(q4) + sin(q1)*sfi*cos(q4)) + bx*cfi*cos(q4);
    
    betta = gammax*ax + gammay*ay;
    
  q6 = acos(  bx*(cos(q1)*sin(q4)+sin(q1)*sfi*cos(q4))  +  by*(sin(q1)*sin(q4)-cos(q1)*sfi*cos(q4))  +  bz*(cfi*cos(q4))  );
  if (betta<0)  q6 = -q6; end; 
  
  % --------------------------------------------
  
  Ind1  = abs(q1)/q1max;
  Ind2  = abs(q2)/q2max;
  Ind3  = abs(q3)/q3max;
  Ind4  = abs(q4)/q4max;
  Ind5  = abs(q5)/q5max;
  Ind6  = abs(q6)/q6max;
  Ind7  = abs(q7)/q7max;
  Ind8  = ( 2 - sqrt(ax*ax+ay*ay) - sqrt(rx*rx+ry*ry)/(L2+L3+L4) ) / 2;
  Ind9  = ( q5max - abs(q5) )/ q5max;
  Ind10 = ( q3max - abs(q3)/4.7 )/ q3max;
  
  J = 0;
  J = max (J,Ind1);
  J = max (J,Ind2);
  J = max (J,Ind3);
  J = max (J,Ind4);
  J = max (J,Ind5);
  J = max (J,Ind6);
  J = max (J,Ind7);
  J = max (J,Ind8);
  J = max (J,Ind9);
  J = max (J,Ind10);
 
  MAP(i) = J;
     
  if (i == N)
      q7 = q7min;
      break;
  end  
  q7 = q7 + (q7max-q7min)/N;    
     
end     
  
  M2 = MAP(2);
  M3 = MAP(3);
  M4 = MAP(4);
  M5 = MAP(5);
  M6 = MAP(6);
  M7 = MAP(7);
  M8 = MAP(8);
  M9 = MAP(9);
  M10 = MAP(10);
  M11 = MAP(11);
  M12 = MAP(12);
  M13 = MAP(13);
  M14 = MAP(14);
  M15 = MAP(15);
  M16 = MAP(16);
  M17 = MAP(17);
  M18 = MAP(18);
  M19 = MAP(19);
  M20 = MAP(20);
  M21 = MAP(21);
  M22 = MAP(22);
  M23 = MAP(23);
  M24 = MAP(24);
  M25 = MAP(25);
  M26 = MAP(26);
  M27 = MAP(27);
  M28 = MAP(28);
  M29 = MAP(29);
  M30 = MAP(30);
  M31 = MAP(31);
  M32 = MAP(32);
  M33 = MAP(33);
  M34 = MAP(34);
  M35 = MAP(35);
  M36 = MAP(36);
  M37 = MAP(37);
  M38 = MAP(38);
  M39 = MAP(39);
  M40 = MAP(40);
  
end

== matlab function BFT1/PathFounder_xyz(tau) ==
  data: v input double; x output double; y output double; z output double; num output double; paramdt output double; paramSUM input double; time input double; ax output double; ay output double; az output double; bx output double; by output double; bz output double
function [x,y,z,num,paramdt,ax,ay,az,bx,by,bz] = fcn(v,paramSUM,time)

  pi = 3.14159265358979;

  % reset initial conditions, when -1 change on +1.
  % Отсчет номера рабочего сплайна.
  num = 2;
  for k = 1:1:99
    if (paramSUM>k) num = k+2; end;
  end;
  param = paramSUM - num + 2;
  
    L1 = 0.4;
    L2 = 0.7;
    L3 = 0.7;
    L4 = 0.1;
  
  % =======================================================================
  
  %% Окружность 0.4R с центром в (.)(0;ky;kz) и хитрые спирали.
%  ky = 1.1;       % Окружность: смещение по оси оу.                                    
%  kz = 0.5;       % Окружность: смещение по оси оz.
%  R  = 0.45;      % Окружность: радиус окружности.
%
%  H  = 1.1;       % Спирали: смещение по oy.
%  J  = 0.25;      % Спирали: смещение по oz.
%  L  = 0.41;      % Спирали: ширина петель по ox.
%  Y  = (L2*cos(pi/6)+L3+L4-0.01);   % Точка сингулярности №2.
%  Z  = L1+L2*sin(pi/6);             % Точка сингулярности №2.
%
  % Положение РИ.
%  Px   = [-R  0    R   0    -R  0    R   0          -3*L -L 0       0        L  3*L       0    -R  0    R   0    -R  0    R   ];
%  Py   = [ky  ky   ky  ky   ky  ky   ky  ky         H    H  1.02*Y  1.025*Y  H  H         ky   ky  ky   ky  ky   ky  ky   ky  ]; 
%  Pz   = [kz  kz-R kz  kz+R kz  kz-R kz  kz+R       J    J  1.02*Z  1.025*Z  J  J         kz+R kz  kz-R kz  kz+R kz  kz-R kz  ];
%
  % Ориентация РИ.
%  Pksi  = [0 0 0 0 0 0 0 0   0 0 0 0 0 0   0 0 0 0 0 0 0 0];
%  Pteta = [0 0 0 0 0 0 0 0   0 0 0 0 0 0   0 0 0 0 0 0 0 0]; 
%  Pfi   = [0 0 0 0 0 0 0 0   0 0 0 0 0 0   0 0 0 0 0 0 0 0];  
  
  % ======================================================================

%  %% Траектория для ТПОМО-2017: спираль.
%  R = 10;
%  h = 30;
%  
%   % Положение РИ.
%  Px   = [0      R      0      -R     0      R      0      -R     0      R      0       -R      0      ];
%  Py   = [R      0      -R     0      R      0      -R     0      R      0      -R      0       R      ];
%  Pz   = [0*h/12 1*h/12 2*h/12 3*h/12 4*h/12 5*h/12 6*h/12 7*h/12 8*h/12 9*h/12 10*h/12 11*h/12 12*h/12];
%
%  % Ориентация РИ.
%  Pksi  = [0 0 0 0 0 0 0 0];
%  Pteta = [0 0 0 0 0 0 0 0]; 
%  Pfi   = [0 0 0 0 0 0 0 0];   

  % =======================================================================
  
  %% Траектория для демонстрации входа в ограничения отдельных степеней подвижности.
  
  % q5=0
  Xsing3  = 0;
  Ysing3  = L2*cos(pi/6)+L3+L4;
  Zsing3  = L1+L2*sin(pi/6);
  kssing3 = 0;
  tesing3 = 0;
  fising3 = 0;
  % sat(q2) и q5=0 
  Xsat2  = 0;
  Ysat2  = L3+L4;
  Zsat2  = L1+L2;
  kssat2 = 0;
  tesat2 = 0;
  fisat2 = 0;
  % sat(q3)
  Xsat3  = ((L2+L4)*pi/4)*sin(pi/10)*0.75;
  Ysat3  = ((L2+L4)*pi/4)*cos(pi/10)*0.75;
  Zsat3  = L1-L3*0.5;%-L4*pi/4;
  kssat3 = 0;%-pi/4;
  tesat3 = 0;
  fisat3 = 0;  
  % sat(q2) 
  Xsat4  = 0;
  Ysat4  = L3+L4;
  Zsat4  = L1+L2;
  kssat4 = -pi/3;
  tesat4 = 0;
  fisat4 = 0;
  % Точка вне досягаемости манипулятора.
  Xsat5  = L2+L3*0.7;
  Ysat5  = L2+0.4*L3;
  Zsat5  = 0;
  kssat5 = 0;
  tesat5 = 0;
  fisat5 = 0;  
  
  % Положение РИ.
  Px   = [Xsing3-0.6 Xsing3-0.3 Xsing3-0.1 Xsing3 Xsing3 Xsing3+0.1 Xsing3+0.3 Xsing3+0.6               Xsat2-0.6 Xsat2-0.4 Xsat2 Xsat2 Xsat2+0.4 Xsat2+0.6               Xsat3-0.1 Xsat3 Xsat3 Xsat3+0.1                Xsat4-0.3 Xsat4-0.1 Xsat4 Xsat4 Xsat4+0.1 Xsat4+0.3         Xsat5 Xsat5+0.2 Xsat5     Xsat5-0.2 Xsat5 Xsat5 ];
  Py   = [Ysing3-0.4 Ysing3-0.3 Ysing3-0.1 Ysing3 Ysing3 Ysing3-0.1 Ysing3-0.3 Ysing3-0.4               Ysat2+0.2 Ysat2+0.1 Ysat2 Ysat2 Ysat2+0.1 Ysat2+0.2               Ysat3+0.3 Ysat3 Ysat3 Ysat3+0.3                Ysat4+0.2 Ysat4+0.1 Ysat4 Ysat4 Ysat4+0.1 Ysat4+0.2         Ysat5 Ysat5     Ysat5     Ysat5     Ysat5 Ysat5 ]; 
  Pz   = [Zsing3     Zsing3     Zsing3     Zsing3 Zsing3 Zsing3     Zsing3     Zsing3                   Zsat2     Zsat2     Zsat2 Zsat2 Zsat2     Zsat2                   Zsat3     Zsat3 Zsat3 Zsat3                    Zsat4     Zsat4     Zsat4 Zsat4 Zsat4     Zsat4             Zsat5 Zsat5+0.2 Zsat5+0.4 Zsat5+0.2 Zsat5 Zsat5 ];
  % Ориентация РИ.
  Pksi  = [0 0 0 kssing3 kssing3 0 0 0                                                                  0 0 kssat2 kssat2 0 0                                             0 kssat3 kssat3 0                              0 0 kssat4 kssat4 0 0                                       kssat5 kssat5 kssat5 kssat5 kssat5 kssat5       ];
  Pteta = [0 0 0 tesing3 tesing3 0 0 0                                                                  0 0 tesat2 tesat2 0 0                                             0 tesat3 tesat3 0                              0 0 tesat4 tesat4 0 0                                       kssat5 tesat5 tesat5 tesat5 tesat5 tesat5       ]; 
  Pfi   = [0 0 0 fising3 fising3 0 0 0                                                                  0 0 fisat2 fisat2 0 0                                             0 fisat3 fisat3 0                              0 0 fisat4 fisat4 0 0                                       kssat5 fisat5 fisat5 fisat5 fisat5 fisat5       ];    

  %% ======================================================================

  % Положение РИ.
  % Расчет коэффициентов A,B,C,D.
  Ax = ( -Px(num-1)   + 3*Px(num) - 3*Px(num+1) + Px(num+2) )/6;
  Ay = ( -Py(num-1)   + 3*Py(num) - 3*Py(num+1) + Py(num+2) )/6;
  Az = ( -Pz(num-1)   + 3*Pz(num) - 3*Pz(num+1) + Pz(num+2) )/6;
  Bx = ( 3*Px(num-1)  - 6*Px(num) + 3*Px(num+1)             )/6;
  By = ( 3*Py(num-1)  - 6*Py(num) + 3*Py(num+1)             )/6;
  Bz = ( 3*Pz(num-1)  - 6*Pz(num) + 3*Pz(num+1)             )/6;
  Cx = ( -3*Px(num-1)             + 3*Px(num+1)             )/6;
  Cy = ( -3*Py(num-1)             + 3*Py(num+1)             )/6;
  Cz = ( -3*Pz(num-1)             + 3*Pz(num+1)             )/6;
  Dx = ( Px(num-1)    + 4*Px(num) + Px(num+1)               )/6;
  Dy = ( Py(num-1)    + 4*Py(num) + Py(num+1)               )/6;
  Dz = ( Pz(num-1)    + 4*Pz(num) + Pz(num+1)               )/6;
  
  x = Ax*param^3 + Bx*param^2 + Cx*param + Dx;
  y = Ay*param^3 + By*param^2 + Cy*param + Dy;
  z = Az*param^3 + Bz*param^2 + Cz*param + Dz;
  
  Fx = 3*Ax*param^2+2*Bx*param+Cx;
  Fy = 3*Ay*param^2+2*By*param+Cy;
  Fz = 3*Az*param^2+2*Bz*param+Cz;
  
  % расчет производной параметрического времени_
  paramdt = v/( Fx^2 + Fy^2 + Fz^2 )^(0.5);
  
  %% ======================================================================

  % Ориентация РИ.
  % Расчет коэффициентов A,B,C,D.  
  Aksi  = ( -Pksi(num-1)    + 3*Pksi(num)  - 3*Pksi(num+1)  + Pksi(num+2)  )/6;
  Ateta = ( -Pteta(num-1)   + 3*Pteta(num) - 3*Pteta(num+1) + Pteta(num+2) )/6;
  Afi   = ( -Pfi(num-1)     + 3*Pfi(num)   - 3*Pfi(num+1)   + Pfi(num+2)   )/6;
  Bksi  = ( 3*Pksi(num-1)   - 6*Pksi(num)  + 3*Pksi(num+1)                 )/6;
  Bteta = ( 3*Pteta(num-1)  - 6*Pteta(num) + 3*Pteta(num+1)                )/6;
  Bfi   = ( 3*Pfi(num-1)    - 6*Pfi(num)   + 3*Pfi(num+1)                  )/6;
  Cksi  = ( -3*Pksi(num-1)                 + 3*Pksi(num+1)                 )/6;
  Cteta = ( -3*Pteta(num-1)                + 3*Pteta(num+1)                )/6;
  Cfi   = ( -3*Pfi(num-1)                  + 3*Pfi(num+1)                  )/6;
  Dksi  = ( Pksi(num-1)     + 4*Pksi(num)  + Pksi(num+1)                   )/6;
  Dteta = ( Pteta(num-1)    + 4*Pteta(num) + Pteta(num+1)                  )/6;
  Dfi   = ( Pfi(num-1)      + 4*Pfi(num)   + Pfi(num+1)                    )/6;  
    
  ksi  = Aksi*param^3  + Bksi*param^2  + Cksi*param  + Dksi;
  teta = Ateta*param^3 + Bteta*param^2 + Cteta*param + Dteta;
  fi   = Afi*param^3   + Bfi*param^2   + Cfi*param   + Dfi;
  
%ksi  = 0;
%teta = 0;
%fi   = 0;
  
  Ea = [ 0 ; 1 ; 0 ];
  Eb = [ 0 ; 0 ; 1 ];
  
  % Mx(ksi) - поворот вокруг оси OX на на угол ksi_
  Mxksi  = [ 1         0          0         ; 0       cos(ksi) (-sin(ksi)) ; 0            sin(ksi) cos(ksi) ];
  Myteta = [ cos(teta) 0          sin(teta) ; 0       1        0           ; (-sin(teta)) 0        cos(teta)];
  Mzfi   = [ cos(fi)   (-sin(fi)) 0         ; sin(fi) cos(fi)  0           ; 0            0        1        ];  
  
  a = Mxksi*Myteta*Mzfi*Ea;
  b = Mxksi*Myteta*Mzfi*Eb;
  
  ax = a(1,1);
  ay = a(2,1);
  az = a(3,1);
  bx = b(1,1);
  by = b(2,1);
  bz = b(3,1);
  
end

== matlab function PZK ==
  data: q1 input double; xx output double; xy output double; q2 input double; q3 input double; q4 input double; q5 input double; q6 input double; q7 input double; q8 input double; xz output double; yx output double; yy output double; yz output double; zx output double; zy output double; zz output double; rx output double; ry output double; rz output double; detJ output double
function [xx,xy,xz,yx,yy,yz,zx,zy,zz,rx,ry,rz,detJ] = fcn(q1,q2,q3,q4,q5,q6,q7,q8)

    L1 = 0.4;
    L2 = 0.7;
    L3 = 0.7;
    L4 = 0.1;
    
  % =======================================================================
  
  s1  = sin(q1);
  s2  = sin(q2);
  s3  = sin(q3);
  s4  = sin(q4);
  s5  = sin(q5);
  s6  = sin(q6);  
  c1  = cos(q1);
  c2  = cos(q2);
  c3  = cos(q3);
  c4  = cos(q4);
  c5  = cos(q5);
  c6  = cos(q6);
  sfi = sin(q2+q3);
  cfi = cos(q2+q3);
  
  A1 = [ (-s1) 0     c1    0     ; c1    0  s1 0     ; 0 1 0 L1 ; 0 0 0 1 ];
  A2 = [ c2    (-s2) 0     L2*c2 ; s2    c2 0  L2*s2 ; 0 0 1 0  ; 0 0 0 1 ];
  A3 = [ (-s3) 0     c3    0     ; c3    0  s3 0     ; 0 1 0 0  ; 0 0 0 1 ];
  A4 = [ (-s4) 0     c4    0     ; c4    0  s4 0     ; 0 1 0 L3 ; 0 0 0 1 ];
  A5 = [ (-c5) 0     (-s5) 0     ; (-s5) 0  c5 0     ; 0 1 0 0  ; 0 0 0 1 ];
  A6 = [ c6   (-s6)  0     0     ; s6    c6 0  0     ; 0 0 1 L4 ; 0 0 0 1 ];
  
  T = A1*A2*A3*A4*A5*A6;
  
  xx = T(1,1);
  xy = T(2,1);
  xz = T(3,1);
  yx = T(1,2);
  yy = T(2,2);
  yz = T(3,2);
  zx = T(1,3);
  zy = T(2,3);
  zz = T(3,3);
  rx = T(1,4) + q7;
  ry = T(2,4) + q8;
  rz = T(3,4);
  
  % стр. 202 ("Системы управления подводными роботами" - зеленая книга)
  % | xx yx zx rx |         
  % | xy yy zy ry |         [ xy yy zy ] = B
  % | xz yz zz rz |         [ xz yz zz ] = A
  % | 0  0  0  1  |, где    [ rx ry rz ] = [ x  y  z ]
  
  % ======================================================================= 
  
  % Расчет Якобиана

  J11 = 0;
  J12 = - cos(q6)*(cfi*sin(q5) + sfi*cos(q5)*sin(q4)) - sfi*cos(q4)*sin(q6);
  J13 = - cos(q6)*(cfi*sin(q5) + sfi*cos(q5)*sin(q4)) - sfi*cos(q4)*sin(q6);
  J14 = cfi*cos(q4)*cos(q5)*cos(q6) - cfi*sin(q4)*sin(q6);
  J15 = -cos(q6)*(sfi*cos(q5) + cfi*sin(q4)*sin(q5));
  J16 = sin(q6)*(sfi*sin(q5) - cfi*cos(q5)*sin(q4)) + cfi*cos(q4)*cos(q6);

  J21 = - sin(q5)*(cos(q1)*cos(q4) - sfi*sin(q1)*sin(q4)) - cfi*cos(q5)*sin(q1);
  J22 = - sfi*cos(q1)*cos(q5) - cfi*cos(q1)*sin(q4)*sin(q5);
  J23 = - sfi*cos(q1)*cos(q5) - cfi*cos(q1)*sin(q4)*sin(q5);
  J24 = sin(q5)*(sin(q1)*sin(q4) - sfi*cos(q1)*cos(q4));
  J25 = - cos(q5)*(cos(q4)*sin(q1) + sfi*cos(q1)*sin(q4)) - cfi*cos(q1)*sin(q5);
  J26 = 0;

  J31 = 0;
  J32 = cfi*cos(q5) - sfi*sin(q4)*sin(q5);
  J33 = cfi*cos(q5) - sfi*sin(q4)*sin(q5);
  J34 = cfi*cos(q4)*sin(q5);
  J35 = cfi*cos(q5)*sin(q4) - sfi*sin(q5);
  J36 = 0;

  J41 = L4*(sin(q5)*(cos(q4)*sin(q1) + sfi*cos(q1)*sin(q4)) - cfi*cos(q1)*cos(q5)) - L3*cfi*cos(q1) - L2*cos(q1)*cos(q2);
  J42 = L4*(sfi*cos(q5)*sin(q1) + cfi*sin(q1)*sin(q4)*sin(q5)) + L3*sfi*sin(q1) + L2*sin(q1)*sin(q2);
  J43 = L4*(sfi*cos(q5)*sin(q1) + cfi*sin(q1)*sin(q4)*sin(q5)) + L3*sfi*sin(q1);
  J44 = L4*sin(q5)*(cos(q1)*sin(q4) + sfi*cos(q4)*sin(q1));
  J45 = -L4*(cos(q5)*(cos(q1)*cos(q4) - sfi*sin(q1)*sin(q4)) - cfi*sin(q1)*sin(q5));
  J46 = 0;

  J51 = L4*sin(q1)*(sin(q5)*(cos(q4)*sin(q1) + sfi*cos(q1)*sin(q4)) - cfi*cos(q5)) - L3*cfi*sin(q1) - L2*cos(q2)*sin(q1) - L4*cos(q1)*sin(q5)*(cos(q1)*cos(q4) - sfi*sin(q1)*sin(q4));
  J52 = - L3*sfi*cos(q1) - L2*cos(q1)*sin(q2) - L4*cos(q1)*(sfi*cos(q5) + cfi*cos(q1)*sin(q4)*sin(q5));
  J53 = - L3*sfi*cos(q1) - L4*cos(q1)*(sfi*cos(q5) + cfi*cos(q1)*sin(q4)*sin(q5));
  J54 = L4*cos(q1)*sin(q5)*(sin(q1)*sin(q4) - sfi*cos(q1)*cos(q4));
  J55 = -L4*cos(q1)*(cos(q5)*(cos(q4)*sin(q1) + sfi*cos(q1)*sin(q4)) + cfi*sin(q5));
  J56 = 0;

  J61 = 0;
  J62 = L3*cfi + L2*cos(q2) + L4*(cfi*cos(q5) - sfi*sin(q4)*sin(q5));
  J63 = L3*cfi + L4*(cfi*cos(q5) - sfi*sin(q4)*sin(q5));
  J64 = L4*cfi*cos(q4)*sin(q5);
  J65 = -L4*(sfi*sin(q5) - cfi*cos(q5)*sin(q4));
  J66 = 0;
  
  J = [ J11 J12 J13 J14 J15 J16 ; 
        J21 J22 J23 J24 J25 J26 ; 
        J31 J32 J33 J34 J35 J36 ; 
        J41 J42 J43 J44 J45 J46 ; 
        J51 J52 J53 J54 J55 J56 ; 
        J61 J62 J63 J64 J65 J66 ];
    
  detJ = abs( det(J) );
  
end
